simulink model "DR_benchmark_LT"  (R2022b)
settings: Solver=ode45  StartTime=63  StopTime=609  FixedStep=0.01  RelTol=1e-5  AbsTol=1e-8
values from neighbouring files (symbols this model uses):
  ACTIVATE = [0]    [benchmarkinit_ASM3_DR.m]
  Qr_DR = Qin * 1.5    [ASM3_DR_datagen.m]    (also in DR_ASM3_Experiment_New.m; benchmarkinit_ASM3_DR_refactored_new.m; benchmarkinit_ASM3_DR_refactored_new2.m)
  TEMPMODEL = [0]    [benchmarkinit_ASM3_DR.m]
undefined symbols (not defined in the file or in its folder): carb1, carb2, carb3, carb4, carb5, KLa1, KLa2, PAR1, Qin0, Qintr, Qw, SOSAT1, T, VOL1, XINIT1, XINITDELAY
settings Model: Creator=ielulf  LastModifiedBy=aya
settings SolverCC: AutoScaleAbsTol=off  AlgebraicLoopSolver=TrustRegion
settings DataIOCC: SaveFormat=Array  SignalLoggingSaveFormat=ModelDataLogs  SaveOutput=off  ReturnWorkspaceOutputs=off  TimeSaveName=t  SignalLoggingName=sigsOut  OutputOption=SpecifiedOutputTimes  OutputTimes=[63:1/96:609]
settings OptimizationCC: BlockReduction=off  BooleanDataType=off  ExpressionDepthLimit=2147483647  InitFltsAndDblsToZero=on  LifeSpan=inf
settings DebuggingCC: AlgebraicLoopMsg=none  SaveWithParameterizedLinksMsg=none  UnderspecifiedInitializationDetection=Classic  MergeDetectMultiDrivingBlocksExec=none  SignalResolutionControl=TryResolveAllWithWarning  InheritedTsInSrcMsg=none  MultiTaskDSMMsg=warning  MultiTaskCondExecSysMsg=none  FcnCallInpInsideContextMsg=warning  UnconnectedInputMsg=warning  UnconnectedLineMsg=warning  StateNameClashWarn=warning  SFUnexpectedBacktrackingDiag=warning  SFNoUnconditionalDefaultTransitionDiag=warning  SFExecutionAtInitializationDiag=none  SFMachineParentedDataDiag=warning  ArithmeticOperatorsInVariantConditions=warning
settings HardwareCC: ProdBitPerPointer=32  ProdBitPerSizeT=32  ProdBitPerPtrDiffT=32  ProdLargestAtomicFloat=None  ProdIntDivRoundTo=Undefined  ProdEndianess=Unspecified  ProdWordSize=32  ProdHWDeviceType=32-bit Generic  TargetBitPerLong=64  TargetBitPerPointer=64  TargetBitPerSizeT=64  TargetBitPerPtrDiffT=64  TargetLongLongMode=on  TargetIntDivRoundTo=Zero  TargetEndianess=LittleEndian  TargetWordSize=64  TargetHWDeviceType=MATLAB Host  ProdEqTarget=off
settings ModelReferenceCC: PropagateSignalLabelsOutOfModel=off
settings RTWCC: TemplateMakefile=grt_unix.tmf
settings CodeAppCC: StateflowObjectComments=on
settings GRTTargetCC: TargetFcnLib=ansi_tfl_tmw.mat  TargetLangStandard=C89/C90 (ANSI)  CombineOutputUpdateFcns=off  GRTInterface=on
settings ConfigComp: CovMetricSettings=dw  CovSaveCumulativeToWorkspaceVar=on  CovSaveSingleToWorkspaceVar=on

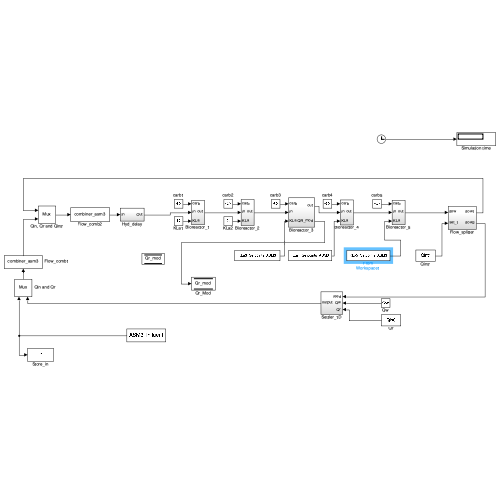
[thumbnail: Simulink's stored preview of the top-level diagram]
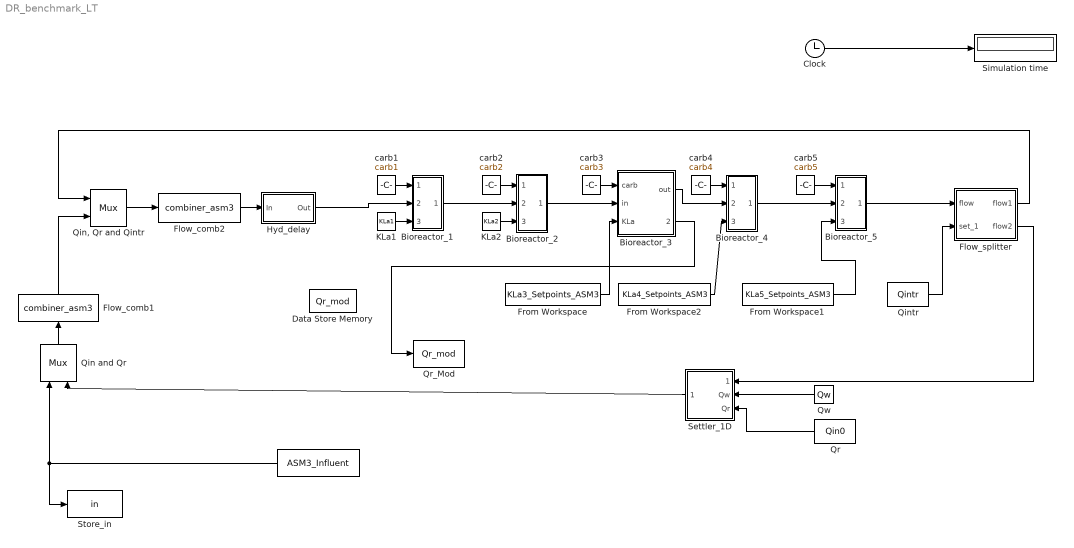
== system DR_benchmark_LT ==
  " " : FromWorkspace  VariableName=ASM3_Influent  SampleTime=-1  ZeroCross=off  OutputAfterFinalValue=Holding final value
  Bioreactor_1 : Subsystem
  Bioreactor_2 : Subsystem
  Bioreactor_3 : Subsystem
  Bioreactor_4 : Subsystem
  Bioreactor_5 : Subsystem
  Clock : Clock
  Data Store Memory : DataStoreMemory  DataStoreName=Qr_mod  WriteAfterWriteMsg=warning  InitialValue=1  ShowAdditionalParam=off
  Flow_comb1 : S-Function  FunctionName=combiner_asm3  SFunctionDeploymentMode=off  EnableBusSupport=off
  Flow_comb2 : S-Function  FunctionName=combiner_asm3  SFunctionDeploymentMode=off  EnableBusSupport=off
  Flow_splitter : Subsystem
  From Workspace : FromWorkspace  VariableName=KLa3_Setpoints_ASM3
  From Workspace1 : FromWorkspace  VariableName=KLa5_Setpoints_ASM3
  From Workspace2 : FromWorkspace  VariableName=KLa4_Setpoints_ASM3
  Hyd_delay : Subsystem
  KLa1 : Constant  Value=KLa1
  KLa2 : Constant  Value=KLa2
  Qin and Qr : Mux  Inputs=2
  "Qin, Qr and Qintr" : Mux  Inputs=2
  Qintr : Constant  Value=Qintr
  Qr : Constant  Value=Qin0
  Qr_Mod : DataStoreWrite  DataStoreName=Qr_mod  IndexOptions=Index vector (dialog)  Indices=1  OutputSizes=1
  Qw : Constant  Value=Qw
  Settler_1D : Subsystem
  Simulation time : Display
  Store_in : ToWorkspace  VariableName=in  SampleTime=-1
  carb1 : Constant  Value=carb1
  carb2 : Constant  Value=carb2
  carb3 : Constant  Value=carb3
  carb4 : Constant  Value=carb4
  carb5 : Constant  Value=carb5
  wires:
  Qin and Qr/1 -> Flow_comb1/1
  "Qin, Qr and Qintr"/1 -> Flow_comb2/1
  Settler_1D/1(output) -> Qin and Qr/2
  Qw/1 -> Settler_1D/2(Qw)
  Bioreactor_5/1(out) -> Flow_splitter/1(flow)
  Clock/1 -> Simulation time/1
  carb1/1 -> Bioreactor_1/1(carb)
  KLa1/1 -> Bioreactor_1/3(KLa)
  Bioreactor_1/1(out) -> Bioreactor_2/2(in)
  KLa2/1 -> Bioreactor_2/3(KLa)
  carb2/1 -> Bioreactor_2/1(carb)
  Bioreactor_2/1(out) -> Bioreactor_3/2(in)
  From Workspace/1 -> Bioreactor_3/3(KLa)
  carb3/1 -> Bioreactor_3/1(carb)
  Bioreactor_3/1(out) -> Bioreactor_4/2(in)
  From Workspace2/1 -> Bioreactor_4/3(KLa)
  carb4/1 -> Bioreactor_4/1(carb)
  Bioreactor_4/1(out) -> Bioreactor_5/2(in)
  carb5/1 -> Bioreactor_5/1(carb)
  From Workspace1/1 -> Bioreactor_5/3(KLa)
  Qintr/1 -> Flow_splitter/2(set_1)
  Flow_comb1/1 -> "Qin, Qr and Qintr"/2
  Flow_comb2/1 -> Hyd_delay/1(In)
  Hyd_delay/1(Out) -> Bioreactor_1/2(in)
  Flow_splitter/1(flow1) -> "Qin, Qr and Qintr"/1
  Flow_splitter/2(flow2) -> Settler_1D/1(feed)
  " "/1 -> Qin and Qr/1, Store_in/1
  Bioreactor_3/2(QR_mod) -> Qr_Mod/1
  Qr/1 -> Settler_1D/3(Qr)

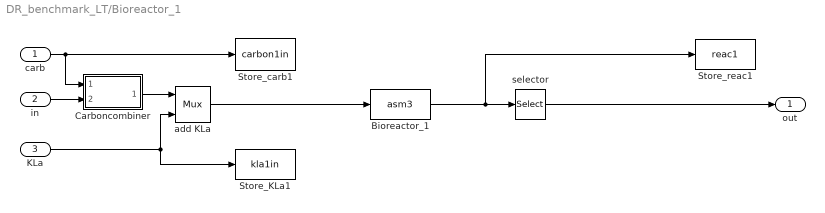
== system DR_benchmark_LT/Bioreactor_1 ==
  carb : Inport
  in : Inport  Port=2
  KLa : Inport  Port=3
  Bioreactor_1 : S-Function  FunctionName=asm3  Parameters=XINIT1,PAR1,VOL1,SOSAT1,TEMPMODEL,ACTIVATE  SFunctionDeploymentMode=off  EnableBusSupport=off
  Carboncombiner : Subsystem
  Store_KLa1 : ToWorkspace  VariableName=kla1in  SampleTime=-1
  Store_carb1 : ToWorkspace  VariableName=carbon1in  SampleTime=-1
  Store_reac1 : ToWorkspace  VariableName=reac1  SampleTime=-1
  add KLa : Mux  Inputs=2
  selector : Selector  InputPortWidth=24  IndexOptions=Index vector (dialog)  Indices=[1 2 3 4 5 6 7 8 9 10 11 12 13 14 15 16 17 18 19 20]  OutputSizes=1
  out : Outport
  wires:
  add KLa/1 -> Bioreactor_1/1
  Bioreactor_1/1 -> Store_reac1/1, selector/1
  Carboncombiner/1(Output) -> add KLa/1
  carb/1 -> Store_carb1/1, Carboncombiner/1(C_flow)
  in/1 -> Carboncombiner/2(Input)
  KLa/1 -> add KLa/2, Store_KLa1/1
  selector/1 -> out/1

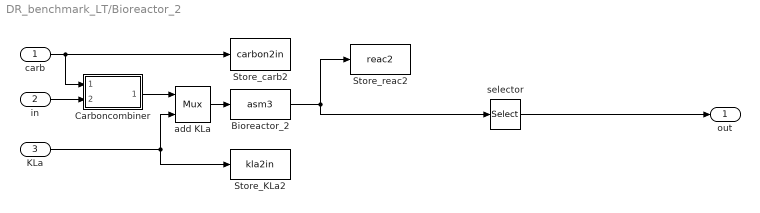
== system DR_benchmark_LT/Bioreactor_2 ==
  carb : Inport
  in : Inport  Port=2
  KLa : Inport  Port=3
  Bioreactor_2 : S-Function  FunctionName=asm3  Parameters=XINIT2,PAR2,VOL2,SOSAT2, TEMPMODEL,ACTIVATE  SFunctionDeploymentMode=off  EnableBusSupport=off
  Carboncombiner : Subsystem
  Store_KLa2 : ToWorkspace  VariableName=kla2in  SampleTime=-1
  Store_carb2 : ToWorkspace  VariableName=carbon2in  SampleTime=-1
  Store_reac2 : ToWorkspace  VariableName=reac2  SampleTime=-1
  add KLa : Mux  Inputs=2
  selector : Selector  InputPortWidth=24  IndexOptions=Index vector (dialog)  Indices=[1 2 3 4 5 6 7 8 9 10 11 12 13 14 15 16 17 18 19 20]  OutputSizes=1
  out : Outport
  wires:
  Bioreactor_2/1 -> Store_reac2/1, selector/1
  add KLa/1 -> Bioreactor_2/1
  Carboncombiner/1(Output) -> add KLa/1
  carb/1 -> Store_carb2/1, Carboncombiner/1(C_flow)
  in/1 -> Carboncombiner/2(Input)
  KLa/1 -> add KLa/2, Store_KLa2/1
  selector/1 -> out/1

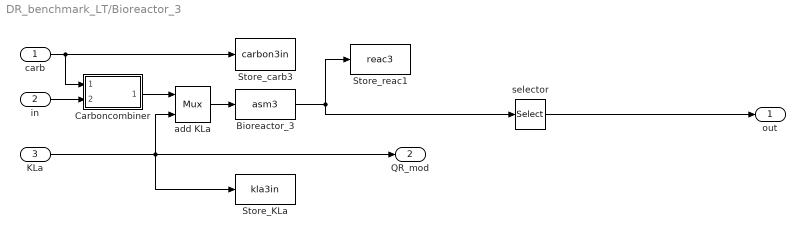
== system DR_benchmark_LT/Bioreactor_3 ==
  carb : Inport
  in : Inport  Port=2
  KLa : Inport  Port=3
  Bioreactor_3 : S-Function  FunctionName=asm3  Parameters=XINIT3,PAR3,VOL3,SOSAT3, TEMPMODEL,ACTIVATE  SFunctionDeploymentMode=off  EnableBusSupport=off
  Carboncombiner : Subsystem
  Store_KLa : ToWorkspace  VariableName=kla3in  SampleTime=-1
  Store_carb3 : ToWorkspace  VariableName=carbon3in  SampleTime=-1
  Store_reac1 : ToWorkspace  VariableName=reac3  SampleTime=-1
  add KLa : Mux  Inputs=2
  selector : Selector  InputPortWidth=24  IndexOptions=Index vector (dialog)  Indices=[1 2 3 4 5 6 7 8 9 10 11 12 13 14 15 16 17 18 19 20]  OutputSizes=1
  out : Outport
  QR_mod : Outport  Port=2
  wires:
  Bioreactor_3/1 -> Store_reac1/1, selector/1
  add KLa/1 -> Bioreactor_3/1
  Carboncombiner/1(Output) -> add KLa/1
  carb/1 -> Store_carb3/1, Carboncombiner/1(C_flow)
  in/1 -> Carboncombiner/2(Input)
  KLa/1 -> QR_mod/1, Store_KLa/1, add KLa/2
  selector/1 -> out/1

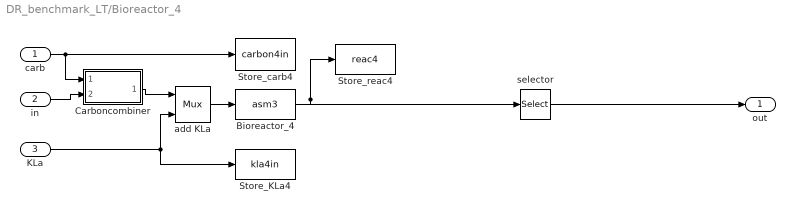
== system DR_benchmark_LT/Bioreactor_4 ==
  carb : Inport
  in : Inport  Port=2
  KLa : Inport  Port=3
  Bioreactor_4 : S-Function  FunctionName=asm3  Parameters=XINIT4,PAR4,VOL4,SOSAT4, TEMPMODEL,ACTIVATE  SFunctionDeploymentMode=off  EnableBusSupport=off
  Carboncombiner : Subsystem
  Store_KLa4 : ToWorkspace  VariableName=kla4in  SampleTime=-1
  Store_carb4 : ToWorkspace  VariableName=carbon4in  SampleTime=-1
  Store_reac4 : ToWorkspace  VariableName=reac4  SampleTime=-1
  add KLa : Mux  Inputs=2
  selector : Selector  InputPortWidth=24  IndexOptions=Index vector (dialog)  Indices=[1 2 3 4 5 6 7 8 9 10 11 12 13 14 15 16 17 18 19 20]  OutputSizes=1
  out : Outport
  wires:
  Bioreactor_4/1 -> Store_reac4/1, selector/1
  add KLa/1 -> Bioreactor_4/1
  Carboncombiner/1(Output) -> add KLa/1
  carb/1 -> Store_carb4/1, Carboncombiner/1(C_flow)
  in/1 -> Carboncombiner/2(Input)
  KLa/1 -> add KLa/2, Store_KLa4/1
  selector/1 -> out/1

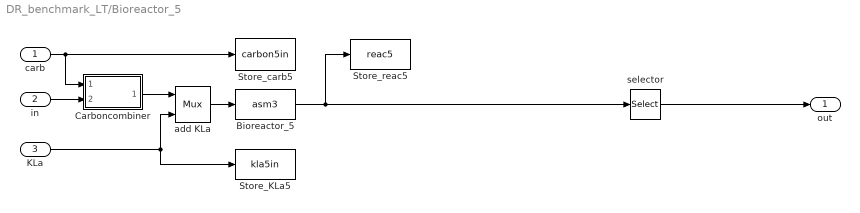
== system DR_benchmark_LT/Bioreactor_5 ==
  carb : Inport
  in : Inport  Port=2
  KLa : Inport  Port=3
  Bioreactor_5 : S-Function  FunctionName=asm3  Parameters=XINIT5,PAR5,VOL5,SOSAT5, TEMPMODEL,ACTIVATE  SFunctionDeploymentMode=off  EnableBusSupport=off
  Carboncombiner : Subsystem
  Store_KLa5 : ToWorkspace  VariableName=kla5in  SampleTime=-1
  Store_carb5 : ToWorkspace  VariableName=carbon5in  SampleTime=-1
  Store_reac5 : ToWorkspace  VariableName=reac5  SampleTime=-1
  add KLa : Mux  Inputs=2
  selector : Selector  InputPortWidth=24  IndexOptions=Index vector (dialog)  Indices=[1 2 3 4 5 6 7 8 9 10 11 12 13 14 15 16 17 18 19 20]  OutputSizes=1
  out : Outport
  wires:
  Bioreactor_5/1 -> Store_reac5/1, selector/1
  add KLa/1 -> Bioreactor_5/1
  Carboncombiner/1(Output) -> add KLa/1
  carb/1 -> Store_carb5/1, Carboncombiner/1(C_flow)
  in/1 -> Carboncombiner/2(Input)
  KLa/1 -> add KLa/2, Store_KLa5/1
  selector/1 -> out/1

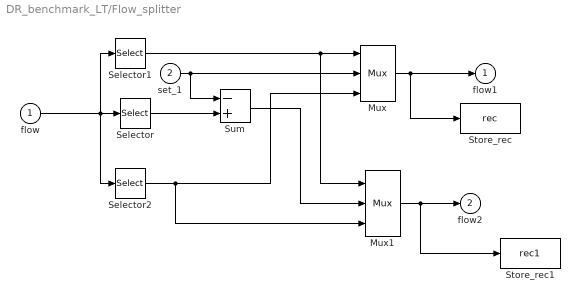
== system DR_benchmark_LT/Flow_splitter ==
  flow : Inport
  set_1 : Inport  Port=2
  Mux : Mux  Inputs=3
  Mux1 : Mux  Inputs=3
  Selector : Selector  InputPortWidth=20  IndexOptions=Index vector (dialog)  Indices=[14]  OutputSizes=1
  Selector1 : Selector  InputPortWidth=20  IndexOptions=Index vector (dialog)  Indices=[1 2 3 4 5 6 7 8 9 10 11 12 13 ]  OutputSizes=1
  Selector2 : Selector  InputPortWidth=20  IndexOptions=Index vector (dialog)  Indices=[15 16 17 18 19 20]  OutputSizes=1
  Store_rec : ToWorkspace  VariableName=rec  SampleTime=-1
  Store_rec1 : ToWorkspace  VariableName=rec1  SampleTime=-1
  Sum : Sum  Inputs=-+  InputSameDT=on  SaturateOnIntegerOverflow=on  OutDataTypeStr=Inherit: Same as first input
  flow1 : Outport
  flow2 : Outport  Port=2
  wires:
  flow/1 -> Selector/1, Selector2/1, Selector1/1
  Mux/1 -> flow1/1, Store_rec/1
  Mux1/1 -> flow2/1, Store_rec1/1
  set_1/1 -> Mux/2, Sum/1
  Selector/1 -> Sum/2
  Sum/1 -> Mux1/2
  Selector1/1 -> Mux/1, Mux1/1
  Selector2/1 -> Mux/3, Mux1/3

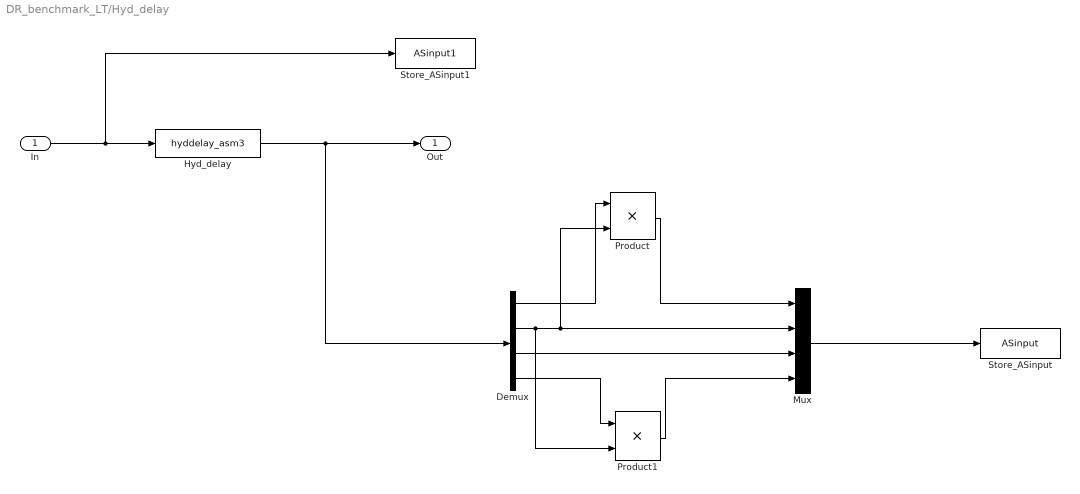
== system DR_benchmark_LT/Hyd_delay ==
  In : Inport
  Demux : Demux  Outputs=[13,1,1,5]
      settings: DisplayOption=none
  Hyd_delay : S-Function  FunctionName=hyddelay_asm3  Parameters=XINITDELAY,PAR1,T  SFunctionDeploymentMode=off  EnableBusSupport=off
  Mux : Mux
  Product : Product  SaturateOnIntegerOverflow=on  OutDataTypeStr=Inherit: Same as first input
  Product1 : Product  SaturateOnIntegerOverflow=on  OutDataTypeStr=Inherit: Same as first input
  Store_ASinput : ToWorkspace  VariableName=ASinput  SampleTime=-1
  Store_ASinput1 : ToWorkspace  VariableName=ASinput1  SampleTime=-1
  Out : Outport
  wires:
  In/1 -> Hyd_delay/1, Store_ASinput1/1
  Hyd_delay/1 -> Out/1, Demux/1
  Demux/1 -> Product/1
  Product/1 -> Mux/1
  Mux/1 -> Store_ASinput/1
  Demux/4 -> Product1/1
  Product1/1 -> Mux/4
  Demux/3 -> Mux/3
  Demux/2 -> Product1/2, Mux/2, Product/2

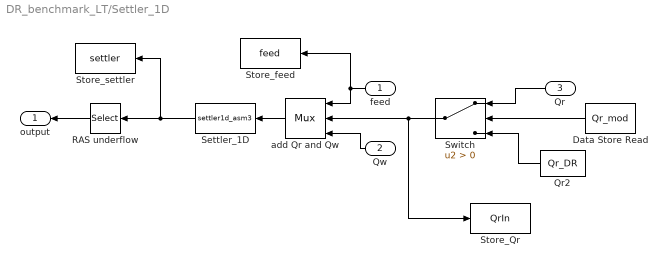
== system DR_benchmark_LT/Settler_1D ==
  feed : Inport
  Qw : Inport  Port=2
  Qr : Inport  Port=3
  Data Store Read : DataStoreRead  DataStoreName=Qr_mod  IndexOptions=Index vector (dialog)  Indices=1  OutputSizes=1
  Qr2 : Constant  Value=Qr_DR
  RAS underflow : Selector  InputPortWidth=243  IndexOptions=Index vector (dialog)  Indices=[1 2 3 4 5 6 7 8 9 10 11 12 13 14 15 16 17 18 19 20]  OutputSizes=1
  Settler_1D : S-Function  FunctionName=settler1d_asm3  Parameters=SETTLERINIT,SETTLERPAR,DIM,LAYER,TEMPMODEL,ACTIVATE, PAR_ASM3, SETTLER  SFunctionDeploymentMode=off  EnableBusSupport=off
  Store_Qr : ToWorkspace  VariableName=QrIn  SampleTime=-1
  Store_feed : ToWorkspace  VariableName=feed  SampleTime=-1
  Store_settler : ToWorkspace  VariableName=settler  SampleTime=-1
  Switch : Switch  Criteria=u2 > Threshold  SaturateOnIntegerOverflow=off  InputSameDT=off
  add Qr and Qw : Mux  Inputs=3
  output : Outport
  wires:
  add Qr and Qw/1 -> Settler_1D/1
  Switch/1 -> Store_Qr/1, add Qr and Qw/2
  Qw/1 -> add Qr and Qw/3
  feed/1 -> add Qr and Qw/1, Store_feed/1
  RAS underflow/1 -> output/1
  Settler_1D/1 -> RAS underflow/1, Store_settler/1
  Qr2/1 -> Switch/3
  Data Store Read/1 -> Switch/2
  Qr/1 -> Switch/1

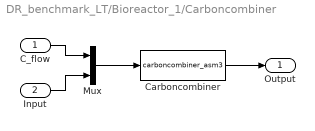
== system DR_benchmark_LT/Bioreactor_1/Carboncombiner ==
  C_flow : Inport
  Input : Inport  Port=2
  Carboncombiner : S-Function  FunctionName=carboncombiner_asm3  Parameters=CARBONSOURCECONC  SFunctionDeploymentMode=off  EnableBusSupport=off
  Mux : Mux  Inputs=2
  Output : Outport
  wires:
  C_flow/1 -> Mux/1
  Mux/1 -> Carboncombiner/1
  Carboncombiner/1 -> Output/1
  Input/1 -> Mux/2

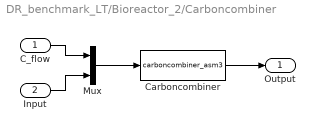
== system DR_benchmark_LT/Bioreactor_2/Carboncombiner ==
  C_flow : Inport
  Input : Inport  Port=2
  Carboncombiner : S-Function  FunctionName=carboncombiner_asm3  Parameters=CARBONSOURCECONC  SFunctionDeploymentMode=off  EnableBusSupport=off
  Mux : Mux  Inputs=2
  Output : Outport
  wires:
  C_flow/1 -> Mux/1
  Mux/1 -> Carboncombiner/1
  Carboncombiner/1 -> Output/1
  Input/1 -> Mux/2

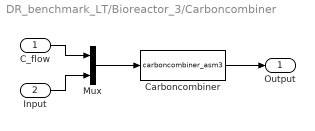
== system DR_benchmark_LT/Bioreactor_3/Carboncombiner ==
  C_flow : Inport
  Input : Inport  Port=2
  Carboncombiner : S-Function  FunctionName=carboncombiner_asm3  Parameters=CARBONSOURCECONC  SFunctionDeploymentMode=off  EnableBusSupport=off
  Mux : Mux  Inputs=2
  Output : Outport
  wires:
  C_flow/1 -> Mux/1
  Mux/1 -> Carboncombiner/1
  Carboncombiner/1 -> Output/1
  Input/1 -> Mux/2

== system DR_benchmark_LT/Bioreactor_4/Carboncombiner ==
  C_flow : Inport
  Input : Inport  Port=2
  Carboncombiner : S-Function  FunctionName=carboncombiner_asm3  Parameters=CARBONSOURCECONC  SFunctionDeploymentMode=off  EnableBusSupport=off
  Mux : Mux  Inputs=2
  Output : Outport
  wires:
  C_flow/1 -> Mux/1
  Mux/1 -> Carboncombiner/1
  Carboncombiner/1 -> Output/1
  Input/1 -> Mux/2

== system DR_benchmark_LT/Bioreactor_5/Carboncombiner ==
  C_flow : Inport
  Input : Inport  Port=2
  Carboncombiner : S-Function  FunctionName=carboncombiner_asm3  Parameters=CARBONSOURCECONC  SFunctionDeploymentMode=off  EnableBusSupport=off
  Mux : Mux  Inputs=2
  Output : Outport
  wires:
  C_flow/1 -> Mux/1
  Mux/1 -> Carboncombiner/1
  Carboncombiner/1 -> Output/1
  Input/1 -> Mux/2
